simulink model "MotGenEvMapped"  (R2023b)
settings: Solver=VariableStepAuto  StartTime=0.0  StopTime=inf  RelTol=1e-3  EnableMultiTasking=on
model workspace (MAT data in the model file):
  EV_current = 200
  EV_motion = [20 4 0.8]
  EV_sf = 2000
  Fs = 0
  Fv = 0.0025
  Jcomp = 0.0227
  Ki = 251.3274
  Kisa = 346.6583
  Kp_d = 0.47149
  Kp_q = 0.52125
  Ksa = 85.4316
  Ksf = 1996.2651
  Ld = 0.0003752
  Ldq = [0.0003752 0.0004148]
  Lq = 0.0004148
  Mechanical = [0.0227 0.0025 0]
  P = 4
  PolePairs = 4
  Rs = 0.2
  T_eff_bp = [0 32.1428571429 64.2857142857 96.4285714286 128.571428571 160.714285714 192.857142857 225 257.142857143 289.285714286 321.428571429 353.571428571 385.714285714 417.857142857 450]
  T_max = 120
  T_mtpa = [0 13.3131834767 26.6278836885 39.9456159322 53.2678926341 66.5962219318 79.9321062746 93.277041051 106.632513247 120.000000141]
  Tc = 0.02
  ba = 3.4029
  efficiency_table = [86.7  86.7  86.7  86.7  86.7  86.7  86.7  86.7  86.7  86.7  86.7  86.7  86.7  86.7  86.7; 86.7  86.7  86.7  86.7  86.7  86.7  86.7  86.7  86.7  86.7  86.7  86.7  86.7  86.7  86.7; 86.7  86.7  91.8  91.8  91.8  91.8  91.8  91.8  91.8  91.8  89.76  89.76  89.76  89.76  89.76; 86.7  86.7  93.84  93.84  93.84  93.84  93.84  93.84  93.84  93.84  93.84  91.8  91.8  91.8  91.8; 86.7  86.7  93.84  93.84  94.86  94.86  94.86  94.86  93.84  93.84  93.84  91.8  91.8  91.8  91.8; 86.7  86.7  94.86  95.88  95.88  95.88  95.88  95.88  95.88  95.88  95.88  95.88  95.88  95.88  95.88; 86.7  86.7  94.86  95.88  95.88  96.9  96.9  96.9  96.9  96.9  96.9  96.9  96.9  96.9  96.9; 86.7  86.7  94.86  95.88  95.88  96.9  96.9  96.9  96.9  96.9  96.9  96.9  96.9  96.9  96.9; 86.7  86.7  94.86  95.88  96.9  96.9  96.9  96.9  96.9  96.9  96.9  96.9  96.9  96.9  96.9; 86.7  86.7  94.86  95.88  96.9  96.9  96.9  96.9  96.9  96.9  96.9  96.9  96.9  96.9  96.9; 86.7  86.7  94.86  95.88  95.88  95.88  95.88  95.88  95.88  95.88  95.88  95.88  95.88  95.88  95.88; 86.7  86.7  91.8  93.84  94.86  94.86  94.86  94.86  94.86  94.86  94.86  94.86  94.86  94.86  94.86]
  id_mtpa = [0 -0.114523352646 -0.457989076459 -1.03008464374 -1.83029075221 -2.85788367342 -4.11193850568 -5.59133329791 -7.29475400168 -9.22070020138]
  idq0 = [0 0]
  idq_limits = [-9.220699542 166.993501392 167.247872355]
  iq_mtpa = [0 18.5827440345 37.1633719111 55.7397734896 74.3098506185 92.871523015 111.422734008 129.961456105 148.485696337 166.993501356]
  lambda_pm = 0.1194
  losses_table = [0  0  0  0  0  0  0  0  0  0  0  0  0  0  0; 0  0  0  0  0  0  0  0  0  0  0  0  0  0  0; 0  0  0  0  0  0  0  0  0  0  0  0  0  0  0; 0  0  0  0  0  0  0  0  0  0  0  0  0  0  0; 0  0  0  0  0  0  0  0  0  0  0  0  0  0  0; 0  0  0  0  0  0  0  0  0  0  0  0  0  0  0; 0  0  0  0  0  0  0  0  0  0  0  0  0  0  0; 0  0  0  0  0  0  0  0  0  0  0  0  0  0  0; 0  0  0  0  0  0  0  0  0  0  0  0  0  0  0; 0  0  0  0  0  0  0  0  0  0  0  0  0  0  0; 0  0  0  0  0  0  0  0  0  0  0  0  0  0  0; 0  0  0  0  0  0  0  0  0  0  0  0  0  0  0]
  mechanical = [0.0227 0.0025 0]
  omega_init = 0
  power_max = 211000
  theta_init = 0
  torque_max = 450
  w_eff_bp = [0 1600 3200 4477.56 4800 6400 8000 9600 11200 12800 14400 16000]
libraries: autolibmappedmotor x1
settings Model: ModifiedByFormat=The MathWorks, Inc.  SimulationMode=accelerator  PauseTimes=10  Creator=The MathWorks, Inc.  LastModifiedBy=The MathWorks, Inc.
settings SolverCC: AlgebraicLoopSolver=TrustRegion  MaxZcPerStep=1
settings DataIOCC: DSMLogging=off  ReturnWorkspaceOutputs=off
settings DebuggingCC: UnderspecifiedInitializationDetection=Classic  MergeDetectMultiDrivingBlocksExec=none  UnconnectedInputMsg=warning  UnconnectedOutputMsg=warning  UnconnectedLineMsg=warning  PregeneratedLibrarySubsystemCodeDiagnostic=none  SubsystemReferenceDiagnosticForUnitTest=warning  ArithmeticOperatorsInVariantConditions=warning
settings ModelReferenceCC: EnableRefExpFcnMdlSchedulingChecks=on  PropagateSignalLabelsOutOfModel=off
settings SFSimCC: SimUseLocalCustomCode=off  CustomCodeUndefinedFunction=UseInterfaceOnly
settings RTWCC: RTWUseLocalCustomCode=off  DLArmComputeVersion=19.05
settings CodeAppCC: StateflowObjectComments=on
settings GRTTargetCC: TargetLangStandard=C89/C90 (ANSI)
settings ConfigComp: CovMetricSettings=dsw  CovSaveCumulativeToWorkspaceVar=on  CovSaveSingleToWorkspaceVar=on  CovExternalEMLEnable=off
settings SimscapeCC: SimscapeNormalizeSystem=off

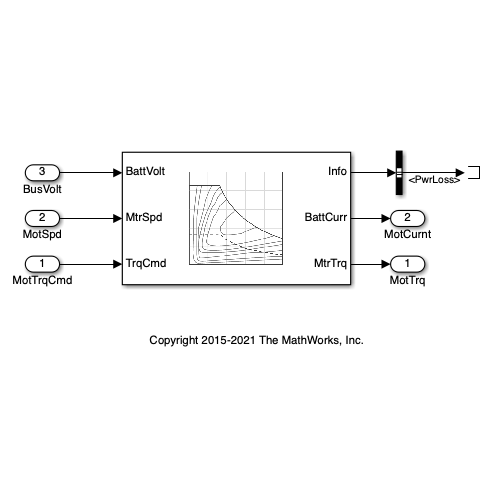
[thumbnail: Simulink's stored preview of the top-level diagram]
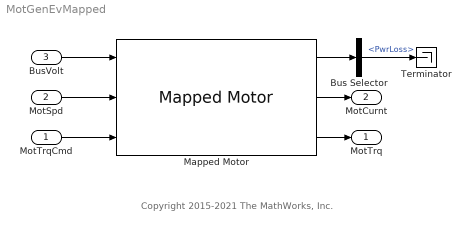
== system MotGenEvMapped ==
  note: Copyright 2015-2021 The MathWorks, Inc.
  MotTrqCmd : Inport
  MotSpd : Inport  Port=2
  BusVolt : Inport  Port=3
  Bus Selector : BusSelector  OutputSignals=PwrLoss
  Mapped Motor : autolibmappedmotor/Mapped Motor  port_config=Speed  param_by=Maximum torque and power  w_t=[ 0 375 750 800 ]  T_t=[0.09 0.08 0.07 0]  torque_max=torque_max  power_max=power_max  Tc=Tc  param_loss=Tabulated efficiency data  eff=100  w_eff=375  T_eff=0.08  Piron=0  Pbase=0  w_eff_bp=w_eff_bp.*pi/30  T_eff_bp=T_eff_bp  Temp_eff_bp=[233.15 293.15 373.15]  losses_table=losses_table  losses_table_3d=cat(3,losses_table,losses_table,losses_table)  efficiency_table=efficiency_table  efficiency_table_3d=cat(3,efficiency_table,efficiency_table,efficiency_table)  J=5e-6  b=1e-5  omega_o=0  T_t_extended=[0 0.07 0.08 0.09 0.08 0.07 0]  w_t_extended=[-800 -750 -375 0 375 750 800]  KLossIron=0  KLossCopper=0  x_w_eff_vec=[-1675.51608191456 -1507.9644737231 -1340.41286553165 -1172.86125734019 -1005.30964914873 -837.758040957278 -670.206432765823 -502.654824574367 -468.888986733584 -335.103216382911 -167.551608191456 0 167.551608191456 335.103216382911 468.888986733584 502.654824574367 670.206432765823 837.758040957278 1005.30964914873 1172.86125734019 1340.41286553165 1507.9644737231 1675.51608191456]  x_T_eff_vec=[-450 -417.857142857143 -385.714285714286 -353.571428571429 -321.428571428571 -289.285714285714 -257.142857142857 -225 -192.857142857143 -160.714285714286 -128.571428571429 -96.4285714285714 -64.2857142857143 -32.1428571428571 0 32.1428571428571 64.2857142857143 96.4285714285714 128.571428571429 160.714285714286 192.857142857143 225 257.142857142857 289.285714285714 321.428571428571 353.571428571429 385.714285714286 417.857142857143 450]  x_tmp_eff_vec=[233.15 293.15 373.15]  x_losses_mat=[40854.6141415599 37936.4274171628 35018.2406927657 32100.0539683685 29181.8672439714 26263.6805195742 23345.4937951771 20427.30707078 17509.1203463828 14590.9336219857 11672.7468975886 10605.888242298 9621.31083452336 8261.6277395441 0 7162.83125018473 8832.36334609244 9952.56552657246 11072.7677070525 13840.9596338156 16609.1515605787 19377.3434873418 22145.535414105 24913.7273408681 27681.9192676312 30450.1111943943 33218.3031211574 35986.4950479206 38754.6869746837;29159.0126646081 27076.2260457076 24993.439426807 22910.6528079064 20827.8661890058 18745.0795701052 16662.2929512047 14579.5063323041 12496.7197134035 10413.9330945029 8331.14647560233 6248.35985670175 5252.73610391485 7435.46496558969 0 6446.54812516626 4982.74546817362 5990.92743060563 7987.90324080751 9984.87905100939 11981.8548612113 13978.8306714131 15975.806481615 17972.7822918169 19969.7581020188 21966.7339122207 23963.7097224225 25960.6855326244 27957.6613428263;19296.9654016165 17918.6107300724 16540.2560585284 15161.9013869844 13783.5467154403 12405.1920438963 11026.8373723523 9648.48270080824 8270.1280292642 6891.77335772017 5513.41868617614 5554.09765040155 4669.09875903542 6609.30219163528 0 5730.26500014778 4429.10708282099 5325.26882720501 5342.50270690469 6678.12838363086 8013.75406035703 9349.3797370832 10685.0054138094 12020.6310905355 13356.2567672617 14691.8824439879 16027.5081207141 17363.1337974402 18698.7594741664;16884.8447264144 15678.7843888134 14472.7240512124 13266.6637136113 12060.6033760103 10854.5430384093 9648.48270080824 8442.4223632072 7236.36202560618 6030.30168800515 4824.24135040412 4859.83544410136 4085.46141415599 5783.13941768087 0 5013.98187512931 3875.46869746837 4659.61022380438 4674.6898685416 5843.362335677 7012.0348028124 8180.7072699478 9349.3797370832 10518.0522042186 11686.724671354 12855.3971384894 14024.0696056248 15192.7420727602 16361.4145398956;14472.7240512124 13438.9580475543 12405.1920438963 11371.4260402383 10337.6600365803 9303.89403292223 8270.1280292642 7236.36202560618 6202.59602194815 5168.83001829013 5554.09765040155 4165.57323780116 3501.82406927657 4956.97664372646 0 4297.69875011084 3321.83031211575 3993.95162040376 5325.26882720501 5008.59628772314 6010.31554526777 7012.0348028124 8013.75406035703 9015.47331790166 10017.1925754463 11018.9118329909 12020.6310905355 13022.3503480802 14024.0696056248;12060.6033760103 11199.1317062953 10337.6600365803 9476.18836686523 8614.71669715021 7753.24502743519 6891.77335772017 6030.30168800515 5168.83001829013 4307.35834857511 4628.41470866796 3471.31103150097 2918.18672439714 4130.81386977205 0 3581.41562509236 2768.19192676312 3328.29301700313 4437.72402267084 4173.83023976929 5008.59628772314 5843.362335677 6678.12838363086 7512.89443158471 8347.66047953857 9182.42652749243 10017.1925754463 10851.9586234001 11686.724671354;12959.5611842703 12033.8782425367 11108.1953008031 10182.5123590695 9256.82941733592 8331.14647560233 7405.46353386874 6479.78059213514 5554.09765040155 4628.41470866796 3702.73176693437 2777.04882520078 2334.54937951771 3304.65109581764 0 2865.13250007389 2214.5535414105 2662.6344136025 3550.17921813667 4437.72402267084 5325.26882720501 6212.81363173918 7100.35843627335 7987.90324080751 8875.44804534168 9762.99284987585 10650.53765441 11538.0824589442 12425.6272634784;20204.7527524991 18761.5561273206 17318.359502142 15875.1628769635 10605.888242298 9545.29941806823 8484.71059383843 6128.19212123399 5252.73610391485 4377.28008659571 3501.82406927657 3181.76647268941 2121.17764845961 2478.48832186323 0 2148.84937505542 1990.51310531449 2985.76965797174 3321.83031211575 4152.28789014468 4982.74546817362 5813.20304620255 7962.05242125797 8957.30897391522 9952.56552657246 14573.3995210525 15898.2540229664 17223.1085248803 18547.9630267941;18847.4984863499 17501.2485944678 16154.9987025857 14808.7488107035 9893.43769962166 8904.0939296595 7914.75015969733 6925.40638973516 5936.062619773 4946.71884981083 3957.37507984867 2968.0313098865 ...(+6504 chars)]  x_losses_mat_3d=cat(3,[93 93 93 93 93 93 93 93 93 93 93 92 90 85 85 85 90 92 93 93 93 93 93 93 93 93 93 93 93;94 94 94 94 94 94 94 94 94 94 94 94 93 85 85 85 93 94 94 94 94 94 94 94 94 94 94 94 94;95 95 95 95 95 95 95 95 95 95 95 94 93 85 85 85 93 94 95 95 95 95 95 95 95 95 95 95 95;95 95 95 95 95 95 95 95 95 95 95 94 93 85 85 85 93 94 95 95 95 95 95 95 95 95 95 95 95;95 95 95 95 95 95 95 95 95 95 94 94 93 85 85 85 93 94 94 95 95 95 95 95 95 95 95 95 95;95 95 95 95 95 95 95 95 95 95 94 94 93 85 85 85 93 94 94 95 95 95 95 95 95 95 95 95 95;94 94 94 94 94 94 94 94 94 94 94 94 93 85 85 85 93 94 94 94 94 94 94 94 94 94 94 94 94;90 90 90 90 92 92 92 93 93 93 93 92 92 85 85 85 92 92 93 93 93 93 92 92 92 90 90 90 90;90 90 90 90 92 92 92 92 92 92 92 92 92 85 85 85 92 92 92 92 92 92 92 92 92 90 90 90 90;88 88 88 88 88 90 90 90 90 90 90 90 90 85 85 85 90 90 90 90 90 90 90 90 88 88 88 88 88;85 85 85 85 85 85 85 85 85 85 85 85 85 85 85 85 85 85 85 85 85 85 85 85 85 85 85 85 85;85 85 85 85 85 85 85 85 85 85 85 85 85 85 85 85 85 85 85 85 85 85 85 85 85 85 85 85 85;85 85 85 85 85 85 85 85 85 85 85 85 85 85 85 85 85 85 85 85 85 85 85 85 85 85 85 85 85;88 88 88 88 88 90 90 90 90 90 90 90 90 85 85 85 90 90 90 90 90 90 90 90 88 88 88 88 88;90 90 90 90 92 92 92 92 92 92 92 92 92 85 85 85 92 92 92 92 92 92 92 92 92 90 90 90 90;90 90 90 90 92 92 92 93 93 93 93 92 92 85 85 85 92 92 93 93 93 93 92 92 92 90 90 90 90;94 94 94 94 94 94 94 94 94 94 94 94 93 85 85 85 93 94 94 94 94 94 94 94 94 94 94 94 94;95 95 95 95 95 95 95 95 95 95 94 94 93 85 85 85 93 94 94 95 95 95 95 95 95 95 95 95 95;95 95 95 95 95 95 95 95 95 95 94 94 93 85 85 85 93 94 94 95 95 95 95 95 95 95 95 95 95;95 95 95 95 95 95 95 95 95 95 95 94 93 85 85 85 93 94 95 95 95 95 95 95 95 95 95 95 95;95 95 95 95 95 95 95 95 95 95 95 94 93 85 85 85 93 94 95 95 95 95 95 95 95 95 95 95 95;94 94 94 94 94 94 94 94 94 94 94 94 93 85 85 85 93 94 94 94 94 94 94 94 94 94 94 94 94;93 93 93 93 93 93 93 93 93 93 93 92 90 85 85 85 90 92 93 93 93 93 93 93 93 93 93 93 93],[93 93 93 93 93 93 93 93 93 93 93 92 90 85 85 85 90 92 93 93 93 93 93 93 93 93 93 93 93;94 94 94 94 94 94 94 94 94 94 94 94 93 85 85 85 93 94 94 94 94 94 94 94 94 94 94 94 94;95 95 95 95 95 95 95 95 95 95 95 94 93 85 85 85 93 94 95 95 95 95 95 95 95 95 95 95 95;95 95 95 95 95 95 95 95 95 95 95 94 93 85 85 85 93 94 95 95 95 95 95 95 95 95 95 95 95;95 95 95 95 95 95 95 95 95 95 94 94 93 85 85 85 93 94 94 95 95 95 95 95 95 95 95 95 95;95 95 95 95 95 95 95 95 95 95 94 94 93 85 85 85 93 94 94 95 95 95 95 95 95 95 95 95 95;94 94 94 94 94 94 94 94 94 94 94 94 93 85 85 85 93 94 94 94 94 94 94 94 94 94 94 94 94;90 90 90 90 92 92 92 93 93 93 93 92 92 85 85 85 92 92 93 93 93 93 92 92 92 90 90 90 90;90 90 90 90 92 92 92 92 92 92 92 92 92 85 85 85 92 92 92 92 92 92 92 92 92 90 90 90 90;88 88 88 88 88 90 90 90 90 90 90 90 90 85 85 85 90 90 90 90 90 90 90 90 88 88 88 88 88;85 85 85 85 85 85 85 85 85 85 85 85 85 85 85 85 85 85 85 85 85 85 85 85 85 85 85 85 85;85 85 85 85 85 85 85 85 85 85 85 85 85 85 85 85 85 85 85 85 85 85 85 85 85 85 85 85 85;85 85 85 85 85 85 85 85 85 85 85 85 85 85 85 85 85 85 85 85 85 85 85 85 85 85 85 85 85;88 88 88 88 88 90 90 90 90 90 90 90 90 85 85 85 90 90 90 90 90 90 90 90 88 88 88 88 88;90 90 90 90 92 92 92 92 92 92 92 92 92 85 85 85 92 92 92 92 92 92 92 92 92 90 90 90 90;90 90 90 90 92 92 92 93 93 93 93 92 92 85 85 85 92 92 93 93 93 93 92 92 92 90 90 90 90;94 94 94 94 94 94 94 94 94 94 94 94 93 85 85 85 93 94 94 94 94 94 94 94 94 94 94 94 94;95 95 95 95 95 95 95 95 95 95 94 94 93 85 85 85 93 94 94 95 95 95 95 95 95 95 95 95 95;95 95 95 95 95 95 95 95 95 95 94 94 93 85 85 85 93 94 94 95 95 95 95 95 95 95 95 95 95;95 95 95 95 95 95 95 95 95 95 95 94 93 85 85 85 93 94 95 95 95 95 95 95 95 95 95 95 95;95 95 95 95 95 95 95 95 95 95 95 94 93 85 85 85 93 94 95 95 95 95 95 95 95 95 95 95 95;94 94 94 94 94 94 94 94 94 94 94 94 93 85 85 85 93 94 94 94 94 94 94 94 94 94 94 94 94;93 93 93 93 93 93 93 93 93 93 93 92 90 85 85 85 90 92 93 93 93 93 93 93 93 93 ...(+2012 chars)])  CalLossMapData={}  CalLossWithTempMapData={}  aMode=aMode  RefBlkName='autolibmappedmotor/Mapped Motor'
  Terminator : Terminator
  MotTrq : Outport  VectorParamsAs1DForOutWhenUnconnected=off
  MotCurnt : Outport  Port=2  VectorParamsAs1DForOutWhenUnconnected=off
  wires:
  MotTrqCmd/1 -> Mapped Motor/3
  BusVolt/1 -> Mapped Motor/1
  MotSpd/1 -> Mapped Motor/2
  Mapped Motor/3 -> MotTrq/1
  Mapped Motor/2 -> MotCurnt/1
  Mapped Motor/1 -> Bus Selector/1
  Bus Selector/1 -> Terminator/1  "<PwrLoss>"
